simulink model "SUBSISTEMA_2"  (R2024b)
settings: Solver=VariableStepAuto  StartTime=0.0  StopTime=10.0  RelTol=1e-3
settings Model: Creator=juani  LastModifiedBy=juani

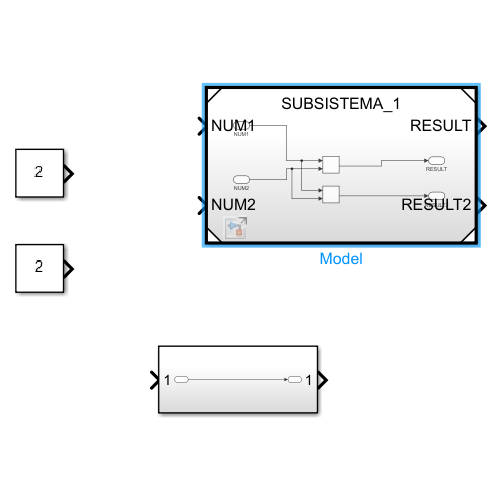
[thumbnail: Simulink's stored preview of the top-level diagram]
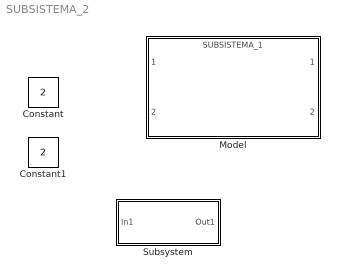
== system SUBSISTEMA_2 ==
  Constant : Constant  Value=2
  Constant1 : Constant  Value=2
  Model : ModelReference  ModelNameDialog=SUBSISTEMA_1.slx  SimulationMode=Normal  ModelReferenceVersion=1.2
  Subsystem : Subsystem

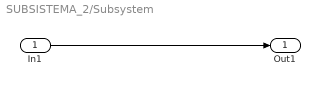
== system SUBSISTEMA_2/Subsystem ==
  In1 : Inport
  Out1 : Outport
  wires:
  In1/1 -> Out1/1
